simulink model "pil_target_mpc5646c_r2015b"  (Simulink 8.6)
settings: Solver=FixedStepDiscrete  StartTime=0.0  StopTime=10.0  RelTol=1e-3
undefined symbols (not defined in the file or in its folder): Newton, Raphson
settings Model: Creator=mbussjaeger  LastModifiedBy=csax
settings OptimizationCC: DefaultParameterBehavior=Inlined  OptimizeModelRefInitCode=on  LifeSpan=1
settings DebuggingCC: FcnCallInpInsideContextMsg=EnableAllAsWarning
settings HardwareCC: ProdIntDivRoundTo=Zero  ProdEndianess=BigEndian  ProdHWDeviceType=Custom Processor->Custom
settings RTWCC: SystemTargetFile=trace32_target_ert.tlc  MakeCommand=trace32_target_make  TemplateMakefile=trace32_mpc_tmf.tmf  Description=TRACE32 Target
settings CodeAppCC: IgnoreCustomStorageClasses=off  MaxIdLength=63
settings STFCustomTargetCC: CombineOutputUpdateFcns=on  ERTCustomFileBanners=on  SupportContinuousTime=off  SupportNonInlinedSFcns=off  MATLABClassNameForMDSCustomization=Simulink.SoftwareTarget.ERTCustomization  GRTInterface=off  SystemTargetFile=trace32_target_ert.tlc
settings ERTTargetCC: MultiwordLength=2048  ParMdlRefBuildCompliant=off  CompOptLevelCompliant=off  ConcurrentExecutionCompliant=off  ERTFirstTimeCompliant=off  ModelStepFunctionPrototypeControlCompliant=off  CPPClassGenCompliant=off  UseToolchainInfoCompliant=off  InlinedParameterPlacement=NonHierarchical  ERTCustomFileTemplate=example_file_process.tlc  ConvertIfToSwitch=off  SuppressUnreachableDefaultCases=off
settings ConfigComp: CovSFcnEnable=off

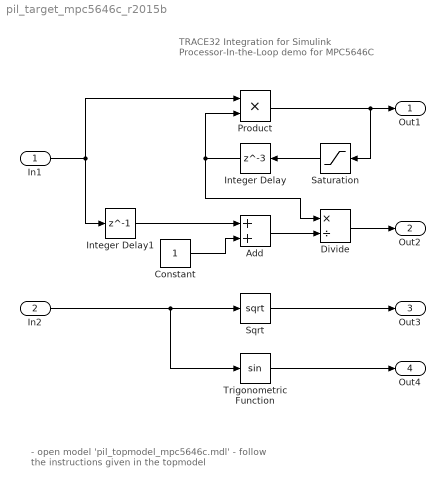
== system pil_target_mpc5646c_r2015b ==
  note: TRACE32 Integration for Simulink
      | Processor-In-the-Loop demo for MPC5646C
  note: - open model 'pil_topmodel_mpc5646c.mdl'
      | - follow the instructions given in the topmodel
  In1 : Inport  OutDataTypeStr=uint16
  In2 : Inport  Port=2  OutDataTypeStr=single
  Add : Sum  AccumDataTypeStr=uint16
  Constant : Constant  OutDataTypeStr=uint16
  Divide : Product  Inputs=*/  OutDataTypeStr=uint16
  Integer Delay : Delay  DelayLength=3  InputProcessing=Inherited
  Integer Delay1 : Delay  DelayLength=1  InputProcessing=Inherited
  Product : Product  OutDataTypeStr=uint16  RndMeth=Zero
  Saturation : Saturate  UpperLimit=6550  LowerLimit=1
  Sqrt : Sqrt  AlgorithmType=Newton-Raphson  SaturateOnIntegerOverflow=on
  Trigonometric Function : Trigonometry
  Out1 : Outport  OutDataTypeStr=uint16
  Out2 : Outport  Port=2  OutDataTypeStr=uint16
  Out3 : Outport  Port=3
  Out4 : Outport  Port=4
  wires:
  In1/1 -> Product/1, Integer Delay1/1
  Saturation/1 -> Integer Delay/1
  Integer Delay/1 -> Product/2, Divide/1
  Product/1 -> Saturation/1, Out1/1
  Divide/1 -> Out2/1
  In2/1 -> Trigonometric Function/1, Sqrt/1
  Sqrt/1 -> Out3/1
  Trigonometric Function/1 -> Out4/1
  Add/1 -> Divide/2
  Constant/1 -> Add/2
  Integer Delay1/1 -> Add/1
